simulink model "Forward_gain_calculation"  (R2019b)
settings: Solver=VariableStepAuto  StartTime=0.0  StopTime=40.0  RelTol=1e-3
undefined symbols (not defined in the file): gamma, k, k0
settings Model: Creator=Mustafa Sezer  LastModifiedBy=Mustafa Sezer

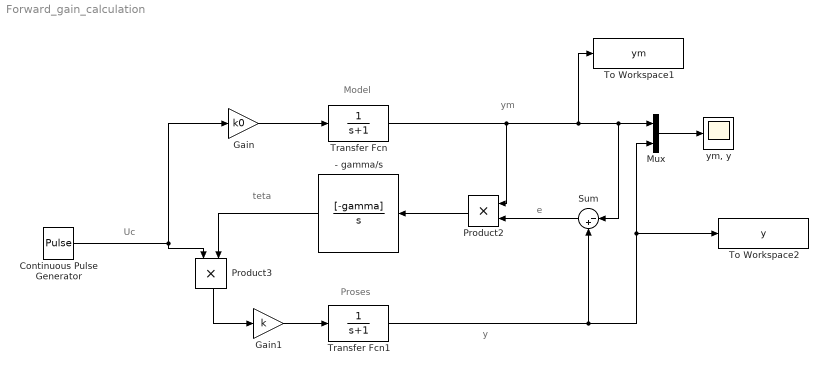
== system Forward_gain_calculation ==
  note: Uc
  note: Model
  note: Proses
  note: e
  note: ym
  note: y
  note: teta
  - gamma/s : TransferFcn  Numerator=[-gamma]  Denominator=[1 0]
  Continuous Pulse Generator : DiscretePulseGenerator  PulseType=Time based  Period=20  PulseWidth=50
  Gain : Gain  Gain=k0
  Gain1 : Gain  Gain=k
  Mux : Mux  Inputs=2
  Product2 : Product
  Product3 : Product
  Sum : Sum  Inputs=|-+
  To Workspace1 : ToWorkspace  VariableName=ym  SaveFormat=Timeseries  SampleTime=-1
  To Workspace2 : ToWorkspace  VariableName=y  SaveFormat=Timeseries  SampleTime=-1
  Transfer Fcn : TransferFcn  Denominator=[1 1]
  Transfer Fcn1 : TransferFcn  Denominator=[1 1]
  "ym, y " : Scope
  wires:
  Continuous Pulse Generator/1 -> Product3/1, Gain/1
  Mux/1 -> "ym, y "/1
  Transfer Fcn/1 -> Product2/1, To Workspace1/1, Sum/1, Mux/1
  Sum/1 -> Product2/2
  Product2/1 -> - gamma/s/1
  - gamma/s/1 -> Product3/2
  Transfer Fcn1/1 -> To Workspace2/1, Mux/2, Sum/2
  Gain/1 -> Transfer Fcn/1
  Gain1/1 -> Transfer Fcn1/1
  Product3/1 -> Gain1/1
